simulink model "PID"  (R2023a)
settings: Solver=VariableStepAuto  StartTime=0.0  StopTime=150  RelTol=1e-3
libraries: cstblocks x2
settings Model: Creator=juan  LastModifiedBy=juan

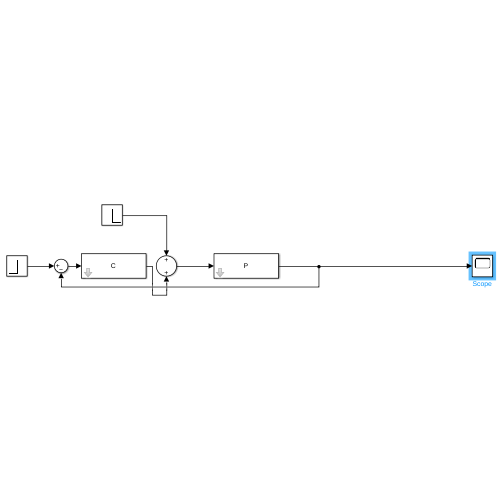
[thumbnail: Simulink's stored preview of the top-level diagram]
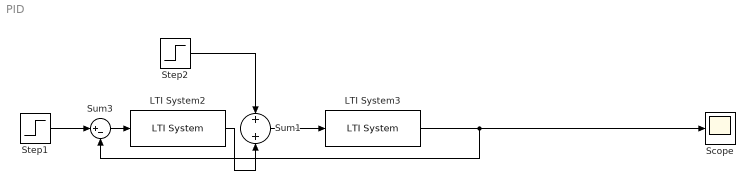
== system PID ==
  LTI System2 : cstblocks/LTI System  sys=C  IC=[]
  LTI System3 : cstblocks/LTI System  sys=P  IC=[]
  Scope : Scope
  Step1 : Step  SampleTime=0
  Step2 : Step  Time=75  After=-0.8  SampleTime=0
  Sum1 : Sum  Inputs=+|+
  Sum3 : Sum  Inputs=|+-
  wires:
  Step2/1 -> Sum1/1
  LTI System2/1 -> Sum1/2
  Step1/1 -> Sum3/1
  Sum3/1 -> LTI System2/1
  Sum1/1 -> LTI System3/1
  LTI System3/1 -> Sum3/2, Scope/1
